simulink model "actuators"  (R2025b)
settings: Solver=VariableStepAuto  StartTime=0.0  StopTime=10.0  RelTol=1e-3
undefined symbols (not defined in the file): tau, w_max
settings Model: Creator=chris  LastModifiedBy=chris
settings ModelReferenceCC: ModelReferenceMinAlgLoopOccurrences=on

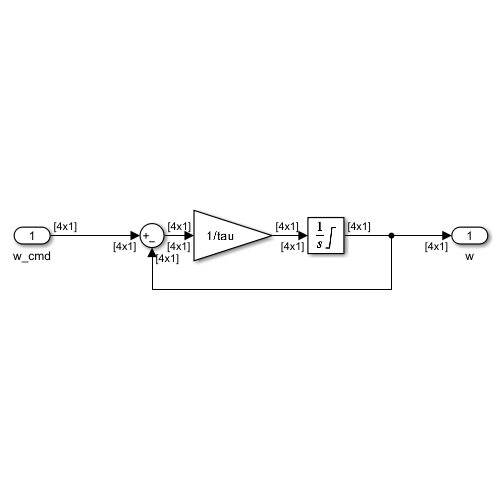
[thumbnail: Simulink's stored preview of the top-level diagram]
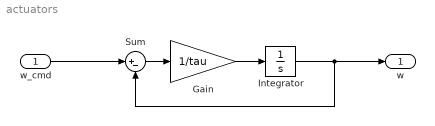
== system actuators ==
  w_cmd : Inport  PortDimensions=[4 1]
  Gain : Gain  Gain=1/tau
  Integrator : Integrator  InitialCondition=zeros(4,1)  LimitOutput=on  UpperSaturationLimit=w_max  LowerSaturationLimit=0
  Sum : Sum  Inputs=|+-
  w : Outport  PortDimensions=[4 1]
  wires:
  Gain/1 -> Integrator/1
  Integrator/1 -> Sum/2, w/1
  w_cmd/1 -> Sum/1
  Sum/1 -> Gain/1
